simulink model "Plant_5"  (R2024b)
settings: Solver=VariableStepAuto  StartTime=0.0  StopTime=2  FixedStep=0.02  RelTol=1e-3
PreLoadFcn:
  | addpath("ref_source\2s\")
model workspace (MAT data in the model file):
  Ref_sig_idx = 2
values from neighbouring files (symbols this model uses):
  A = zeros(4, 4)    [Initialise_var_0.m]
  B = zeros(4, 2)    [Initialise_var_0.m]
  E = [1 0 0 0; 0 1 0 0]    [sfbia.m]    (also in state_feedback_0.m; state_feedback_3.m; state_feedback_4.m)
  Ki = K_aug(:, n+1:end)    [sfbia.m]
  Kx = K_aug(:, 1:n)    [sfbia.m]
  L1 = 0.095    [Initialise_var_0.m]
  L2 = 0.095    [Initialise_var_0.m]
settings Model: Creator=Sez26  LastModifiedBy=Sez26

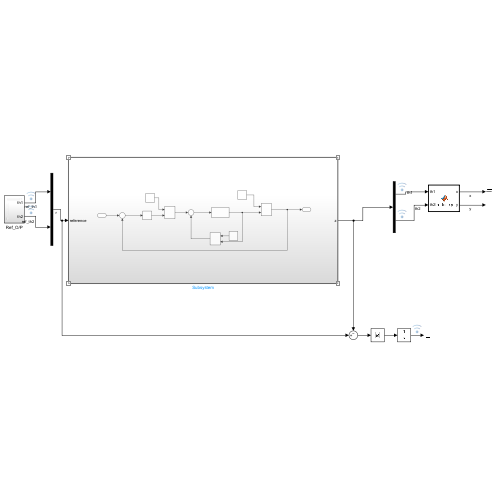
[thumbnail: Simulink's stored preview of the top-level diagram]
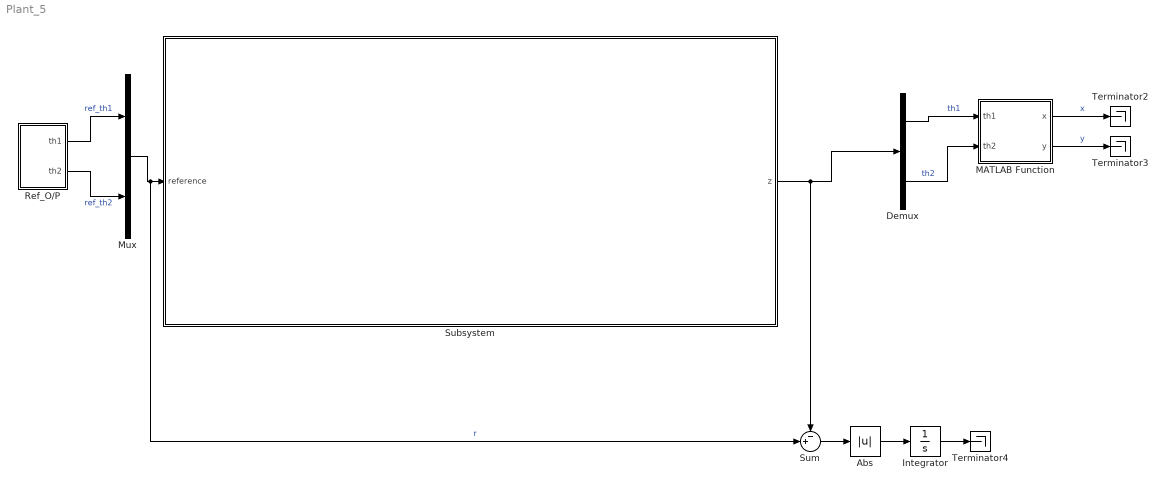
== system Plant_5 ==
  Abs : Abs  SaturateOnIntegerOverflow=off
  Demux : Demux  Outputs=2
  Integrator : Integrator
  MATLAB Function : MATLAB Function  TreatAsAtomicUnit=on
  Mux : Mux  Inputs=2
  Ref_O/P : Subsystem
  Subsystem : Subsystem
  Sum : Sum  Inputs=-+|
  Terminator2 : Terminator
  Terminator3 : Terminator
  Terminator4 : Terminator
  wires:
  MATLAB Function/1(x) -> Terminator2/1  "x"
  MATLAB Function/2(y) -> Terminator3/1  "y"
  Demux/2 -> MATLAB Function/2(th2)  "th2"
  Demux/1 -> MATLAB Function/1(th1)  "th1"
  Ref_O/P/1(th1) -> Mux/1  "ref_th1"
  Ref_O/P/2(th2) -> Mux/2  "ref_th2"
  Mux/1 -> Sum/2, Subsystem/1(reference)  "r"
  Subsystem/1(z) -> Demux/1, Sum/1
  Sum/1 -> Abs/1
  Integrator/1 -> Terminator4/1
  Abs/1 -> Integrator/1

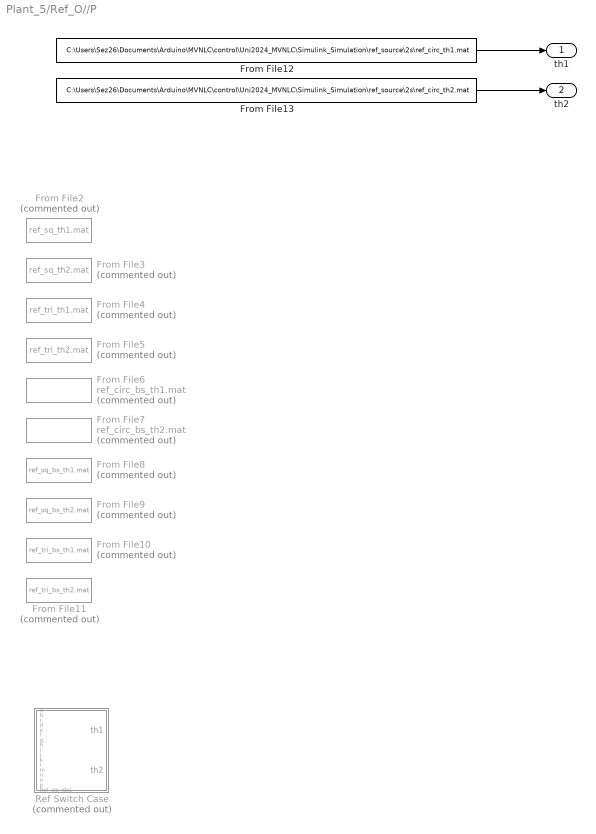
== system Plant_5/Ref_O//P ==
  From File10 : FromFile  Commented=on  FileName=ref_tri_bs_th1.mat  SampleTime=0
  From File11 : FromFile  Commented=on  FileName=ref_tri_bs_th2.mat  SampleTime=0
  From File12 : FromFile  FileName=C:\Users\Sez26\Documents\Arduino\MVNLC\control\Uni2024_MVNLC\Simulink_Simulation\ref_source\2s\ref_circ_th1.mat  SampleTime=0
  From File13 : FromFile  FileName=C:\Users\Sez26\Documents\Arduino\MVNLC\control\Uni2024_MVNLC\Simulink_Simulation\ref_source\2s\ref_circ_th2.mat  SampleTime=0
  From File2 : FromFile  Commented=on  FileName=ref_sq_th1.mat  SampleTime=0
  From File3 : FromFile  Commented=on  FileName=ref_sq_th2.mat  SampleTime=0
  From File4 : FromFile  Commented=on  FileName=ref_tri_th1.mat  SampleTime=0
  From File5 : FromFile  Commented=on  FileName=ref_tri_th2.mat  SampleTime=0
  From File6 : FromFile  Commented=on  FileName=ref_circ_bs_th1.mat  SampleTime=0
  From File7 : FromFile  Commented=on  FileName=ref_circ_bs_th2.mat  SampleTime=0
  From File8 : FromFile  Commented=on  FileName=ref_sq_bs_th1.mat  SampleTime=0
  From File9 : FromFile  Commented=on  FileName=ref_sq_bs_th2.mat  SampleTime=0
  Ref Switch Case : MATLAB Function  Commented=on  TreatAsAtomicUnit=on
  th1 : Outport
  th2 : Outport  Port=2
  wires:
  From File12/1 -> th1/1
  From File13/1 -> th2/1

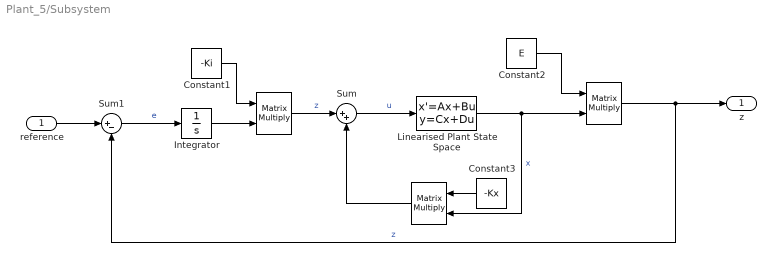
== system Plant_5/Subsystem ==
  reference : Inport
  " " : Product  Multiplication=Matrix(*)
  "  " : Product  Multiplication=Matrix(*)
  "   " : Product  Multiplication=Matrix(*)
  Constant1 : Constant  Value=-Ki
  Constant2 : Constant  Value=E
  Constant3 : Constant  Value=-Kx
  Integrator : Integrator
  Linearised Plant State Space : StateSpace  A=A  B=B  C=[1 0 0 0; 0 1 0 0; 0 0 1 0; 0 0 0 1]  D=[0 0; 0 0; 0 0; 0 0]  InitialCondition=[30, -30, 0 , 0]
  Sum : Sum  Inputs=|++
  Sum1 : Sum  Inputs=|+-
  z : Outport
  wires:
  Constant2/1 -> "  "/1
  Integrator/1 -> " "/2
  Linearised Plant State Space/1 -> "   "/2, "  "/2  "x"
  Sum/1 -> Linearised Plant State Space/1  "u"
  " "/1 -> Sum/1  "z"
  Constant3/1 -> "   "/1
  Constant1/1 -> " "/1
  "  "/1 -> Sum1/2, z/1  "z"
  reference/1 -> Sum1/1
  Sum1/1 -> Integrator/1  "e"
  "   "/1 -> Sum/2

== matlab function Plant_5/Ref_O//P/Ref Switch Case ==
  data: Ref_sig_idx parameter; a input; b input; c input; d input; e input; f input; g input; h input; i input; j input; k input; l input; m input; n input; o input; p input; Ref_sig_idx1 input; th1 output; th2 output
function [th1, th2] = ref_switch(Ref_sig_idx, a, b, c, d, e, f, g, h, i, j, k, l, m, n, o, p, Ref_sig_idx1)
    if Ref_sig_idx == 0
        % circ base
        th1 = a;
        th2 = b;
    elseif Ref_sig_idx == 1
        % sq base
        th1 = c;
        th2 = d;
    elseif Ref_sig_idx == 2
        % tri base
        th1 = e;
        th2 = f;
    end
    if Ref_sig_idx == 3
        % circ b spline
        th1 = g;
        th2 = h;
    elseif Ref_sig_idx == 4
        % sq b spline
        th1 = i;
        th2 = j;
    elseif Ref_sig_idx == 5
        % tri b spline
        th1 = k;
        th2 = l;
    end
    if Ref_sig_idx == 6
        % sq corner sf
        th1 = m;
        th2 = n;
    elseif Ref_sig_idx == 7
        % tri corner sf
        th1 = o;
        th2 = p;
    else
        % invalid reference choice
        disp('Error invalid reference choice')
        th1 = 0;
        th2 = 0;
    end

== matlab function Plant_5/MATLAB Function ==
  data: x output; th1 input; y output; th2 input; L1 parameter; L2 parameter
function [x,y] = th_to_xy(th1, th2, L1, L2)
    x = L1*cos(deg2rad(th1)) + L2*cos(deg2rad(th2));
    y = L1*sin(deg2rad(th1)) + L2*sin(deg2rad(th2));
